simulink subsystem "nplib_sensors"  (R2024b)
settings: Solver=VariableStepAuto  StartTime=0.0  StopTime=10.0  RelTol=1e-3
undefined symbols (not defined in the file): convertTo, datetime
libraries: aerolibconvert2 x7
settings Model: Creator=CETCA  LastModifiedBy=CETCA

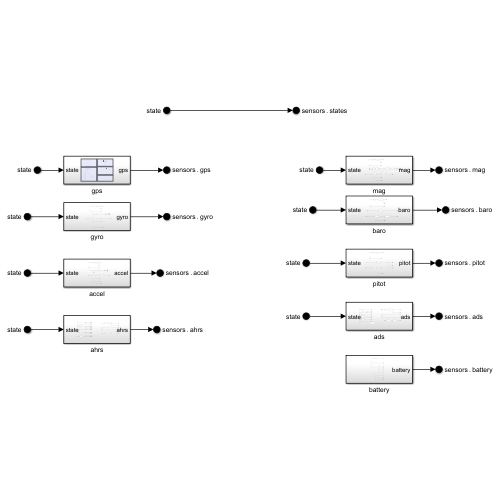
[thumbnail: Simulink's stored preview of the top-level diagram]
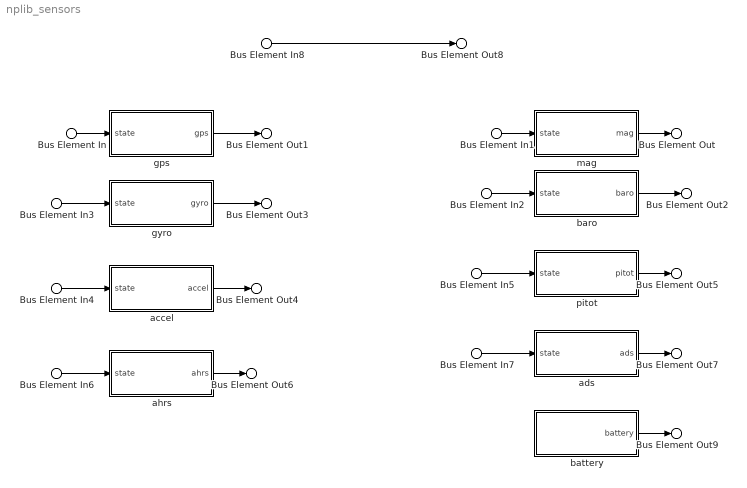
== system nplib_sensors ==
  Bus Element In{,1..8} (9 alike) : Inport  PortName=state
  accel : Subsystem
  ads : Subsystem
  ahrs : Subsystem
  baro : Subsystem
  battery : Subsystem
  gps : Subsystem
  gyro : Subsystem
  mag : Subsystem
  pitot : Subsystem
  Bus Element Out8 : Outport  PortName=sensors  Element=states
  Bus Element Out1 : Outport  PortName=sensors  Element=gps
  Bus Element Out3 : Outport  PortName=sensors  Element=gyro
  Bus Element Out : Outport  PortName=sensors  Element=mag
  Bus Element Out2 : Outport  PortName=sensors  Element=baro
  Bus Element Out5 : Outport  PortName=sensors  Element=pitot
  Bus Element Out7 : Outport  PortName=sensors  Element=ads
  Bus Element Out6 : Outport  PortName=sensors  Element=ahrs
  Bus Element Out4 : Outport  PortName=sensors  Element=accel
  Bus Element Out9 : Outport  PortName=sensors  Element=battery
  wires:
  Bus Element In7/1 -> ads/1(state)
  Bus Element In6/1 -> ahrs/1(state)
  Bus Element In8/1 -> Bus Element Out8/1
  baro/1(baro) -> Bus Element Out2/1
  Bus Element In5/1 -> pitot/1(state)
  mag/1(mag) -> Bus Element Out/1
  battery/1(battery) -> Bus Element Out9/1
  Bus Element In2/1 -> baro/1(state)
  ahrs/1(ahrs) -> Bus Element Out6/1
  Bus Element In1/1 -> mag/1(state)
  pitot/1(pitot) -> Bus Element Out5/1
  accel/1(accel) -> Bus Element Out4/1
  Bus Element In4/1 -> accel/1(state)
  gyro/1(gyro) -> Bus Element Out3/1
  Bus Element In3/1 -> gyro/1(state)
  ads/1(ads) -> Bus Element Out7/1
  Bus Element In/1 -> gps/1(state)
  gps/1(gps) -> Bus Element Out1/1

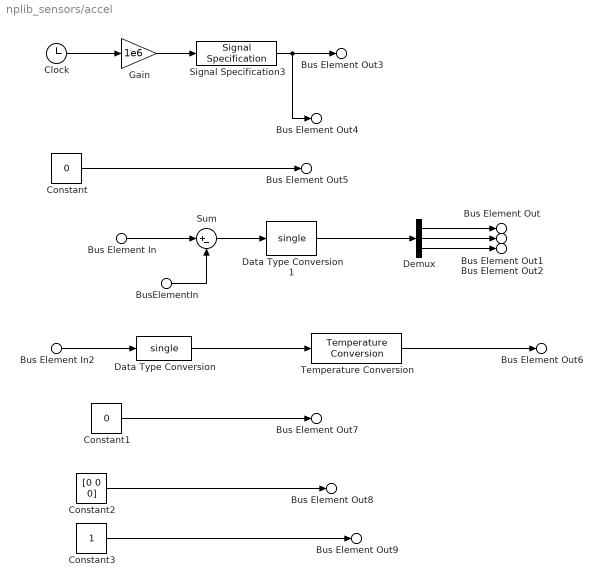
== system nplib_sensors/accel ==
  Bus Element In2 : Inport  PortName=state  Element=environ.atmosphere.temperature
  BusElementIn : Inport  PortName=state  Element=environ.gravity.gx_gy_gz
  Bus Element In : Inport  PortName=state  Element=aircraft.position.ax_ay_az
  Clock : Clock
  Constant : Constant  Value=0  OutDataTypeStr=uint32
  Constant1 : Constant  Value=0  OutDataTypeStr=uint32
  Constant2 : Constant  Value=[0 0 0]  OutDataTypeStr=uint8
  Constant3 : Constant  OutDataTypeStr=uint8
  Data Type Conversion : DataTypeConversion  OutDataTypeStr=single  SaturateOnIntegerOverflow=off  RndMeth=Floor
  Data Type Conversion1 : DataTypeConversion  OutDataTypeStr=single  SaturateOnIntegerOverflow=off  RndMeth=Floor
  Demux : Demux  Outputs=3
  Gain : Gain  Gain=1e6  OutDataTypeStr=uint64
  Signal Specification3 : SignalSpecification  Unit=µs
  Sum : Sum  Inputs=|+-
  Temperature Conversion : aerolibconvert2/Temperature Conversion  IU=K  OU=C
  Bus Element Out3 : Outport  PortName=accel  Element=timestamp
  Bus Element Out4 : Outport  PortName=accel  Element=timestamp_sample
  Bus Element Out5 : Outport  PortName=accel  Element=device_id
  Bus Element Out : Outport  PortName=accel  Element=x
  Bus Element Out1 : Outport  PortName=accel  Element=y
  Bus Element Out2 : Outport  PortName=accel  Element=z
  Bus Element Out6 : Outport  PortName=accel  Element=temperature
  Bus Element Out7 : Outport  PortName=accel  Element=error_count
  Bus Element Out8 : Outport  PortName=accel  Element=clip_counter
  Bus Element Out9 : Outport  PortName=accel  Element=samples
  wires:
  Constant3/1 -> Bus Element Out9/1
  Constant2/1 -> Bus Element Out8/1
  Demux/1 -> Bus Element Out/1
  Demux/2 -> Bus Element Out1/1
  Demux/3 -> Bus Element Out2/1
  Clock/1 -> Gain/1
  Signal Specification3/1 -> Bus Element Out4/1, Bus Element Out3/1
  Gain/1 -> Signal Specification3/1
  Constant/1 -> Bus Element Out5/1
  Constant1/1 -> Bus Element Out7/1
  Bus Element In2/1 -> Data Type Conversion/1
  Temperature Conversion/1 -> Bus Element Out6/1
  Data Type Conversion/1 -> Temperature Conversion/1
  Data Type Conversion1/1 -> Demux/1
  Bus Element In/1 -> Sum/1
  BusElementIn/1 -> Sum/2
  Sum/1 -> Data Type Conversion1/1

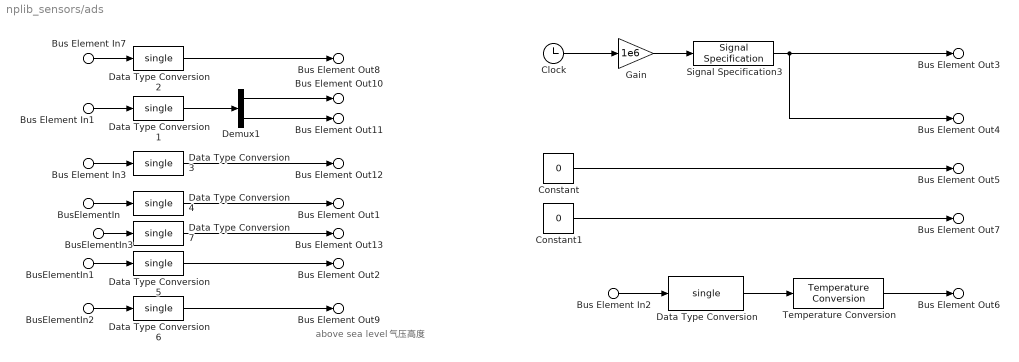
== system nplib_sensors/ads ==
  note: above sea level
      | 气压高度
  Bus Element In2 : Inport  PortName=state  Element=environ.atmosphere.temperature
  BusElementIn : Inport  PortName=state  Element=environ.atmosphere.ps
  BusElementIn1 : Inport  PortName=state  Element=environ.atmosphere.rho
  BusElementIn3 : Inport  PortName=state  Element=environ.atmosphere.pt
  Bus Element In1 : Inport  PortName=state  Element=aircraft.airdata.alpha_beta
  Bus Element In7 : Inport  PortName=state  Element=aircraft.airdata.airspeed
  Bus Element In3 : Inport  PortName=state  Element=aircraft.airdata.qbar
  BusElementIn2 : Inport  PortName=state  Element=aircraft.position.alt
  Clock : Clock
  Constant : Constant  Value=0  OutDataTypeStr=uint32
  Constant1 : Constant  Value=0  OutDataTypeStr=uint32
  Data Type Conversion{,1..7} (8 alike) : DataTypeConversion  OutDataTypeStr=single  SaturateOnIntegerOverflow=off  RndMeth=Floor
  Demux1 : Demux  Outputs=2
  Gain : Gain  Gain=1e6  OutDataTypeStr=uint64
  Signal Specification3 : SignalSpecification  Unit=µs
  Temperature Conversion : aerolibconvert2/Temperature Conversion  IU=K  OU=C
  Bus Element Out3 : Outport  PortName=ads  Element=timestamp
  Bus Element Out4 : Outport  PortName=ads  Element=timestamp_sample
  Bus Element Out5 : Outport  PortName=ads  Element=device_id
  Bus Element Out7 : Outport  PortName=ads  Element=error_count
  Bus Element Out6 : Outport  PortName=ads  Element=temperature
  Bus Element Out8 : Outport  PortName=ads  Element=va
  Bus Element Out10 : Outport  PortName=ads  Element=alpha
  Bus Element Out11 : Outport  PortName=ads  Element=beta
  Bus Element Out12 : Outport  PortName=ads  Element=qbar
  Bus Element Out13 : Outport  PortName=ads  Element=pt
  Bus Element Out1 : Outport  PortName=ads  Element=ps
  Bus Element Out2 : Outport  PortName=ads  Element=rho
  Bus Element Out9 : Outport  PortName=ads  Element=asl
  wires:
  Data Type Conversion3/1 -> Bus Element Out12/1
  Bus Element In3/1 -> Data Type Conversion3/1
  Demux1/2 -> Bus Element Out11/1
  Demux1/1 -> Bus Element Out10/1
  Bus Element In1/1 -> Data Type Conversion1/1
  Clock/1 -> Gain/1
  Signal Specification3/1 -> Bus Element Out4/1, Bus Element Out3/1
  Gain/1 -> Signal Specification3/1
  Constant/1 -> Bus Element Out5/1
  Constant1/1 -> Bus Element Out7/1
  Bus Element In2/1 -> Data Type Conversion/1
  Temperature Conversion/1 -> Bus Element Out6/1
  Data Type Conversion/1 -> Temperature Conversion/1
  Bus Element In7/1 -> Data Type Conversion2/1
  Data Type Conversion1/1 -> Demux1/1
  Data Type Conversion2/1 -> Bus Element Out8/1
  BusElementIn/1 -> Data Type Conversion4/1
  Data Type Conversion4/1 -> Bus Element Out1/1
  BusElementIn1/1 -> Data Type Conversion5/1
  Data Type Conversion5/1 -> Bus Element Out2/1
  BusElementIn2/1 -> Data Type Conversion6/1
  Data Type Conversion6/1 -> Bus Element Out9/1
  Data Type Conversion7/1 -> Bus Element Out13/1
  BusElementIn3/1 -> Data Type Conversion7/1

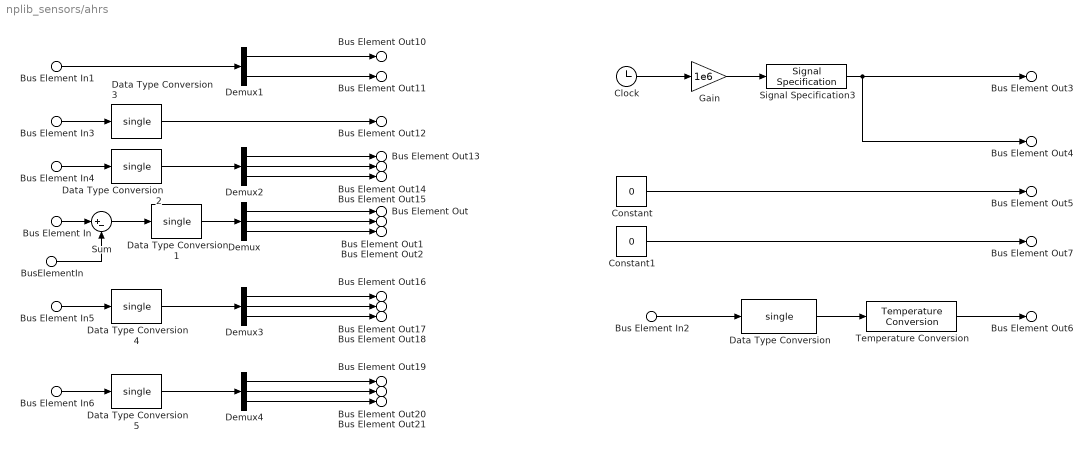
== system nplib_sensors/ahrs ==
  Bus Element In2 : Inport  PortName=state  Element=environ.atmosphere.temperature
  BusElementIn : Inport  PortName=state  Element=environ.gravity.gx_gy_gz
  Bus Element In : Inport  PortName=state  Element=aircraft.position.ax_ay_az
  Bus Element In1 : Inport  PortName=state  Element=aircraft.position.lat_lon
  Bus Element In3 : Inport  PortName=state  Element=aircraft.position.alt
  Bus Element In4 : Inport  PortName=state  Element=aircraft.position.vn_ve_vd
  Bus Element In5 : Inport  PortName=state  Element=aircraft.attitude.phi_theta_psi
  Bus Element In6 : Inport  PortName=state  Element=aircraft.attitude.p_q_r
  Clock : Clock
  Constant : Constant  Value=0  OutDataTypeStr=uint32
  Constant1 : Constant  Value=0  OutDataTypeStr=uint32
  Data Type Conversion{,1..5} (6 alike) : DataTypeConversion  OutDataTypeStr=single  SaturateOnIntegerOverflow=off  RndMeth=Floor
  Demux{,2..4} (4 alike) : Demux  Outputs=3
  Demux1 : Demux  Outputs=2
  Gain : Gain  Gain=1e6  OutDataTypeStr=uint64
  Signal Specification3 : SignalSpecification  Unit=µs
  Sum : Sum  Inputs=|+-
  Temperature Conversion : aerolibconvert2/Temperature Conversion  IU=K  OU=C
  Bus Element Out3 : Outport  PortName=ahrs  Element=timestamp
  Bus Element Out4 : Outport  PortName=ahrs  Element=timestamp_sample
  Bus Element Out5 : Outport  PortName=ahrs  Element=device_id
  Bus Element Out7 : Outport  PortName=ahrs  Element=error_count
  Bus Element Out6 : Outport  PortName=ahrs  Element=temperature
  Bus Element Out10 : Outport  PortName=ahrs  Element=lat
  Bus Element Out11 : Outport  PortName=ahrs  Element=lon
  Bus Element Out12 : Outport  PortName=ahrs  Element=alt
  Bus Element Out13 : Outport  PortName=ahrs  Element=vn
  Bus Element Out14 : Outport  PortName=ahrs  Element=ve
  Bus Element Out15 : Outport  PortName=ahrs  Element=vd
  Bus Element Out : Outport  PortName=ahrs  Element=ax
  Bus Element Out1 : Outport  PortName=ahrs  Element=ay
  Bus Element Out2 : Outport  PortName=ahrs  Element=az
  Bus Element Out16 : Outport  PortName=ahrs  Element=phi
  Bus Element Out17 : Outport  PortName=ahrs  Element=theta
  Bus Element Out18 : Outport  PortName=ahrs  Element=psi
  Bus Element Out19 : Outport  PortName=ahrs  Element=p
  Bus Element Out20 : Outport  PortName=ahrs  Element=q
  Bus Element Out21 : Outport  PortName=ahrs  Element=r
  wires:
  Data Type Conversion1/1 -> Demux/1
  Data Type Conversion/1 -> Temperature Conversion/1
  Temperature Conversion/1 -> Bus Element Out6/1
  Bus Element In2/1 -> Data Type Conversion/1
  Constant1/1 -> Bus Element Out7/1
  Constant/1 -> Bus Element Out5/1
  Gain/1 -> Signal Specification3/1
  Signal Specification3/1 -> Bus Element Out3/1, Bus Element Out4/1
  Clock/1 -> Gain/1
  Demux/3 -> Bus Element Out2/1
  Demux/2 -> Bus Element Out1/1
  Demux/1 -> Bus Element Out/1
  Bus Element In1/1 -> Demux1/1
  Demux1/1 -> Bus Element Out10/1
  Demux1/2 -> Bus Element Out11/1
  Bus Element In3/1 -> Data Type Conversion3/1
  Bus Element In4/1 -> Data Type Conversion2/1
  Demux2/1 -> Bus Element Out13/1
  Demux2/2 -> Bus Element Out14/1
  Demux2/3 -> Bus Element Out15/1
  Bus Element In5/1 -> Data Type Conversion4/1
  Demux3/1 -> Bus Element Out16/1
  Demux3/2 -> Bus Element Out17/1
  Demux3/3 -> Bus Element Out18/1
  Bus Element In6/1 -> Data Type Conversion5/1
  Demux4/1 -> Bus Element Out19/1
  Demux4/2 -> Bus Element Out20/1
  Demux4/3 -> Bus Element Out21/1
  Data Type Conversion2/1 -> Demux2/1
  Data Type Conversion3/1 -> Bus Element Out12/1
  Data Type Conversion4/1 -> Demux3/1
  Data Type Conversion5/1 -> Demux4/1
  Bus Element In/1 -> Sum/1
  Sum/1 -> Data Type Conversion1/1
  BusElementIn/1 -> Sum/2

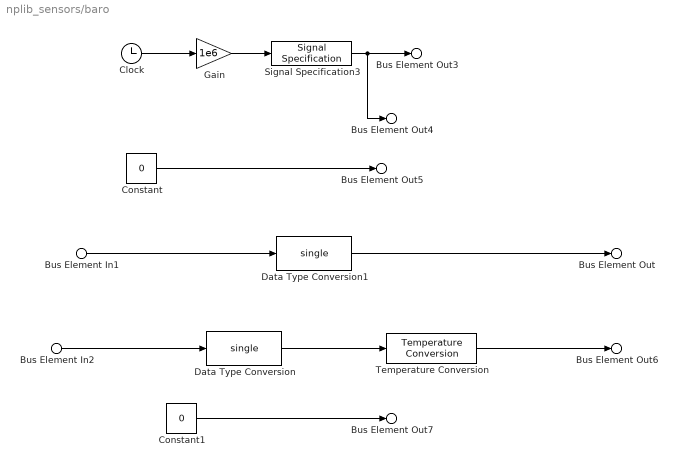
== system nplib_sensors/baro ==
  Bus Element In2 : Inport  PortName=state  Element=environ.atmosphere.temperature
  Bus Element In1 : Inport  PortName=state  Element=environ.atmosphere.ps
  Clock : Clock
  Constant : Constant  Value=0  OutDataTypeStr=uint32
  Constant1 : Constant  Value=0  OutDataTypeStr=uint32
  Data Type Conversion : DataTypeConversion  OutDataTypeStr=single  SaturateOnIntegerOverflow=off  RndMeth=Floor
  Data Type Conversion1 : DataTypeConversion  OutDataTypeStr=single  SaturateOnIntegerOverflow=off  RndMeth=Floor
  Gain : Gain  Gain=1e6  OutDataTypeStr=uint64
  Signal Specification3 : SignalSpecification  Unit=µs
  Temperature Conversion : aerolibconvert2/Temperature Conversion  IU=K  OU=C
  Bus Element Out3 : Outport  PortName=baro  Element=timestamp
  Bus Element Out4 : Outport  PortName=baro  Element=timestamp_sample
  Bus Element Out5 : Outport  PortName=baro  Element=device_id
  Bus Element Out7 : Outport  PortName=baro  Element=error_count
  Bus Element Out : Outport  PortName=baro  Element=pressure
  Bus Element Out6 : Outport  PortName=baro  Element=temperature
  wires:
  Clock/1 -> Gain/1
  Signal Specification3/1 -> Bus Element Out4/1, Bus Element Out3/1
  Gain/1 -> Signal Specification3/1
  Constant/1 -> Bus Element Out5/1
  Constant1/1 -> Bus Element Out7/1
  Bus Element In2/1 -> Data Type Conversion/1
  Temperature Conversion/1 -> Bus Element Out6/1
  Data Type Conversion/1 -> Temperature Conversion/1
  Bus Element In1/1 -> Data Type Conversion1/1
  Data Type Conversion1/1 -> Bus Element Out/1

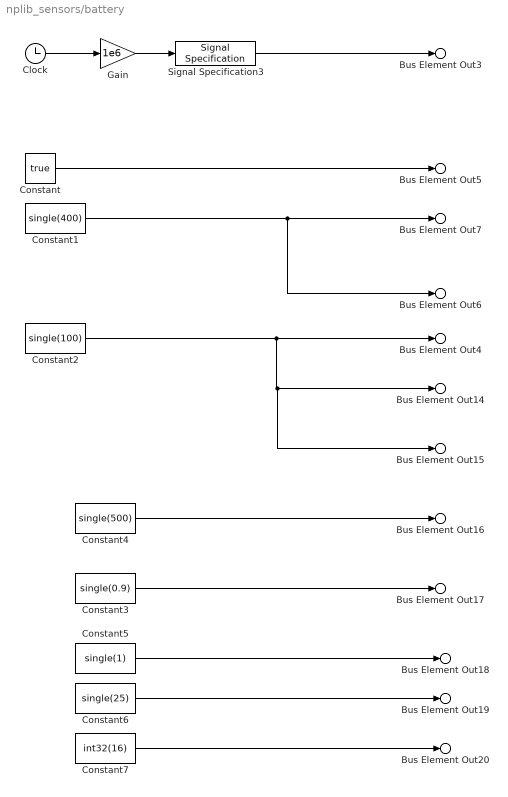
== system nplib_sensors/battery ==
  Clock : Clock
  Constant : Constant  Value=true
  Constant1 : Constant  Value=single(400)
  Constant2 : Constant  Value=single(100)
  Constant3 : Constant  Value=single(0.9)
  Constant4 : Constant  Value=single(500)
  Constant5 : Constant  Value=single(1)
  Constant6 : Constant  Value=single(25)
  Constant7 : Constant  Value=int32(16)
  Gain : Gain  Gain=1e6  OutDataTypeStr=uint64
  Signal Specification3 : SignalSpecification  Unit=µs
  Bus Element Out3 : Outport  PortName=battery  Element=timestamp
  Bus Element Out5 : Outport  PortName=battery  Element=connected
  Bus Element Out7 : Outport  PortName=battery  Element=voltage_v
  Bus Element Out6 : Outport  PortName=battery  Element=voltage_filtered_v
  Bus Element Out4 : Outport  PortName=battery  Element=current_a
  Bus Element Out14 : Outport  PortName=battery  Element=current_filtered_a
  Bus Element Out15 : Outport  PortName=battery  Element=current_average_a
  Bus Element Out16 : Outport  PortName=battery  Element=discharged_mah
  Bus Element Out17 : Outport  PortName=battery  Element=remaining
  Bus Element Out18 : Outport  PortName=battery  Element=scale
  Bus Element Out19 : Outport  PortName=battery  Element=temperature
  Bus Element Out20 : Outport  PortName=battery  Element=cell_count
  wires:
  Constant1/1 -> Bus Element Out6/1, Bus Element Out7/1
  Constant/1 -> Bus Element Out5/1
  Gain/1 -> Signal Specification3/1
  Signal Specification3/1 -> Bus Element Out3/1
  Clock/1 -> Gain/1
  Constant2/1 -> Bus Element Out15/1, Bus Element Out14/1, Bus Element Out4/1
  Constant3/1 -> Bus Element Out17/1
  Constant4/1 -> Bus Element Out16/1
  Constant5/1 -> Bus Element Out18/1
  Constant6/1 -> Bus Element Out19/1
  Constant7/1 -> Bus Element Out20/1

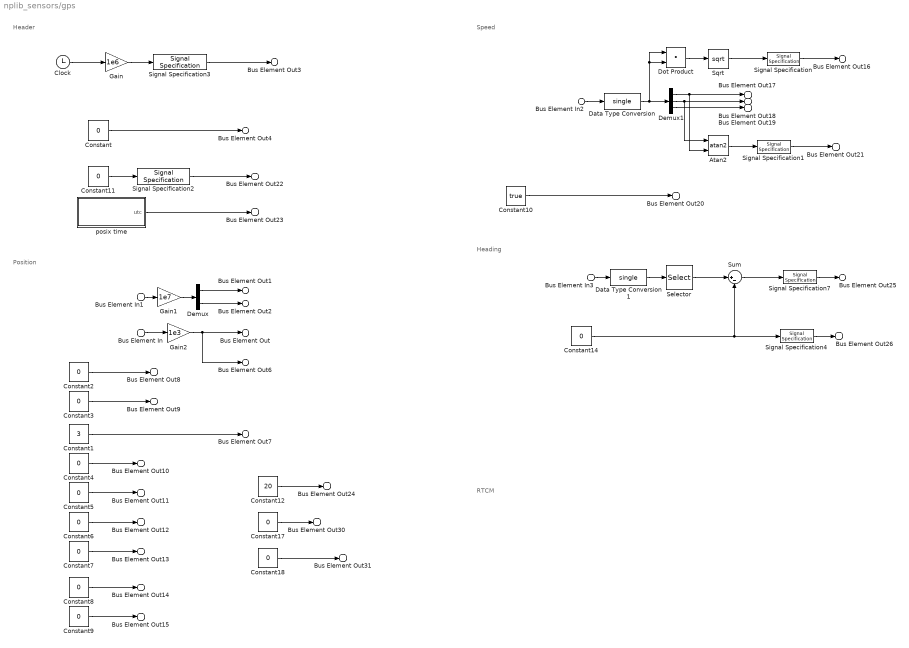
== system nplib_sensors/gps ==
  note: RTCM
  note: Heading
  note: Speed
  note: Header
  note: Position
  Bus Element In : Inport  PortName=state  Element=aircraft.position.alt
  Bus Element In1 : Inport  PortName=state  Element=aircraft.position.lat_lon
  Bus Element In2 : Inport  PortName=state  Element=aircraft.position.vn_ve_vd
  Bus Element In3 : Inport  PortName=state  Element=aircraft.attitude.phi_theta_psi
  Atan2 : Trigonometry  Operator=atan2
  Clock : Clock
  Constant : Constant  Value=0  OutDataTypeStr=uint32
  Constant1 : Constant  Value=3  OutDataTypeStr=uint8
  Constant10 : Constant  Value=true  OutDataTypeStr=boolean
  Constant11 : Constant  Value=0  OutDataTypeStr=int32
  Constant12 : Constant  Value=20  OutDataTypeStr=uint8
  Constant{2..7,14} (7 alike) : Constant  Value=0  OutDataTypeStr=single
  Constant17 : Constant  Value=0  OutDataTypeStr=uint8
  Constant18 : Constant  Value=0  OutDataTypeStr=int32
  Constant8 : Constant  Value=0  OutDataTypeStr=int32
  Constant9 : Constant  Value=0  OutDataTypeStr=uint16
  Data Type Conversion : DataTypeConversion  OutDataTypeStr=single  SaturateOnIntegerOverflow=off  RndMeth=Floor
  Data Type Conversion1 : DataTypeConversion  OutDataTypeStr=single  SaturateOnIntegerOverflow=off  RndMeth=Floor
  Demux : Demux  Outputs=2
  Demux1 : Demux  Outputs=3
  Dot Product : DotProduct  OutDataTypeStr=Inherit: Inherit via internal rule
  Gain : Gain  Gain=1e6  OutDataTypeStr=uint64
  Gain1 : Gain  Gain=1e7  OutDataTypeStr=int32
  Gain2 : Gain  Gain=1e3  OutDataTypeStr=int32
  Selector : Selector  InputPortWidth=3  IndexOptions=Index vector (dialog)  Indices=3  OutputSizes=1
  Signal Specification : SignalSpecification  Unit=m/s
  Signal Specification1 : SignalSpecification  Unit=rad
  Signal Specification2 : SignalSpecification  Unit=ms
  Signal Specification3 : SignalSpecification  Unit=µs
  Signal Specification4 : SignalSpecification  Unit=rad
  Signal Specification7 : SignalSpecification  Unit=rad
  Sqrt : Sqrt
  Sum : Sum  Inputs=|+-
  posix time : Subsystem
  Bus Element Out3 : Outport  PortName=gps  Element=timestamp
  Bus Element Out4 : Outport  PortName=gps  Element=device_id
  Bus Element Out1 : Outport  PortName=gps  Element=lat
  Bus Element Out2 : Outport  PortName=gps  Element=lon
  Bus Element Out : Outport  PortName=gps  Element=alt
  Bus Element Out6 : Outport  PortName=gps  Element=alt_ellipsoid
  Bus Element Out8 : Outport  PortName=gps  Element=s_variance_m_s
  Bus Element Out9 : Outport  PortName=gps  Element=c_variance_rad
  Bus Element Out7 : Outport  PortName=gps  Element=fix_type
  Bus Element Out10 : Outport  PortName=gps  Element=eph
  Bus Element Out11 : Outport  PortName=gps  Element=epv
  Bus Element Out12 : Outport  PortName=gps  Element=hdop
  Bus Element Out13 : Outport  PortName=gps  Element=vdop
  Bus Element Out14 : Outport  PortName=gps  Element=noise_per_ms
  Bus Element Out15 : Outport  PortName=gps  Element=automatic_gain_control
  Bus Element Out31 : Outport  PortName=gps  Element=jamming_indicator
  Bus Element Out30 : Outport  PortName=gps  Element=jamming_state
  Bus Element Out16 : Outport  PortName=gps  Element=vel_m_s
  Bus Element Out17 : Outport  PortName=gps  Element=vel_n_m_s
  Bus Element Out18 : Outport  PortName=gps  Element=vel_e_m_s
  Bus Element Out19 : Outport  PortName=gps  Element=vel_d_m_s
  Bus Element Out21 : Outport  PortName=gps  Element=cog_rad
  Bus Element Out20 : Outport  PortName=gps  Element=vel_ned_valid
  Bus Element Out22 : Outport  PortName=gps  Element=timestamp_time_relative
  Bus Element Out23 : Outport  PortName=gps  Element=time_utc_usec
  Bus Element Out24 : Outport  PortName=gps  Element=satellites_used
  Bus Element Out25 : Outport  PortName=gps  Element=heading
  Bus Element Out26 : Outport  PortName=gps  Element=heading_offset
  wires:
  Bus Element In/1 -> Gain2/1
  Bus Element In1/1 -> Gain1/1
  Demux/1 -> Bus Element Out1/1
  Demux/2 -> Bus Element Out2/1
  Clock/1 -> Gain/1
  Gain/1 -> Signal Specification3/1
  Constant/1 -> Bus Element Out4/1
  Gain1/1 -> Demux/1
  Gain2/1 -> Bus Element Out6/1, Bus Element Out/1
  Constant1/1 -> Bus Element Out7/1
  Constant2/1 -> Bus Element Out8/1
  Constant3/1 -> Bus Element Out9/1
  Constant4/1 -> Bus Element Out10/1
  Constant5/1 -> Bus Element Out11/1
  Constant7/1 -> Bus Element Out13/1
  Constant6/1 -> Bus Element Out12/1
  Constant9/1 -> Bus Element Out15/1
  Constant8/1 -> Bus Element Out14/1
  Bus Element In2/1 -> Data Type Conversion/1
  Demux1/1 -> Atan2/2, Bus Element Out17/1
  Demux1/2 -> Atan2/1, Bus Element Out18/1
  Demux1/3 -> Bus Element Out19/1
  Constant10/1 -> Bus Element Out20/1
  Atan2/1 -> Signal Specification1/1
  Sqrt/1 -> Signal Specification/1
  Dot Product/1 -> Sqrt/1
  Data Type Conversion/1 -> Demux1/1, Dot Product/1, Dot Product/2
  Signal Specification/1 -> Bus Element Out16/1
  Signal Specification1/1 -> Bus Element Out21/1
  Constant12/1 -> Bus Element Out24/1
  Bus Element In3/1 -> Data Type Conversion1/1
  Constant14/1 -> Sum/2, Signal Specification4/1
  Selector/1 -> Sum/1
  Sum/1 -> Signal Specification7/1
  Constant11/1 -> Signal Specification2/1
  posix time/1(utc) -> Bus Element Out23/1
  Signal Specification2/1 -> Bus Element Out22/1
  Signal Specification3/1 -> Bus Element Out3/1
  Signal Specification4/1 -> Bus Element Out26/1
  Constant17/1 -> Bus Element Out30/1
  Constant18/1 -> Bus Element Out31/1
  Signal Specification7/1 -> Bus Element Out25/1
  Data Type Conversion1/1 -> Selector/1

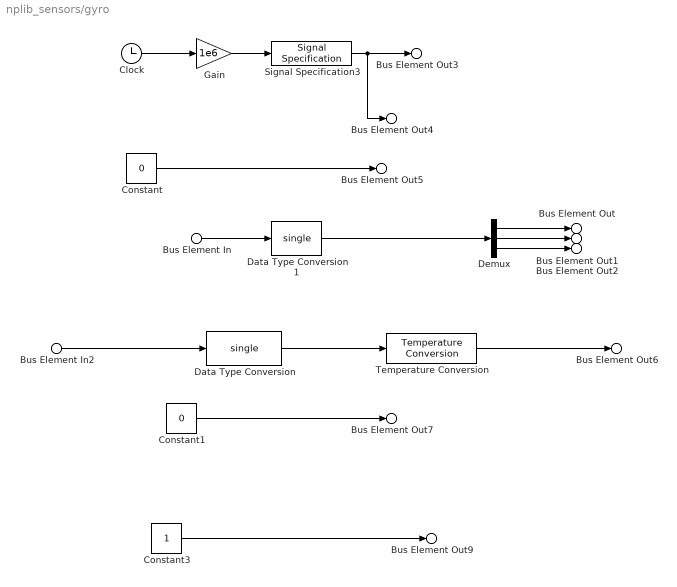
== system nplib_sensors/gyro ==
  Bus Element In2 : Inport  PortName=state  Element=environ.atmosphere.temperature
  Bus Element In : Inport  PortName=state  Element=aircraft.attitude.p_q_r
  Clock : Clock
  Constant : Constant  Value=0  OutDataTypeStr=uint32
  Constant1 : Constant  Value=0  OutDataTypeStr=uint32
  Constant3 : Constant  OutDataTypeStr=uint8
  Data Type Conversion : DataTypeConversion  OutDataTypeStr=single  SaturateOnIntegerOverflow=off  RndMeth=Floor
  Data Type Conversion1 : DataTypeConversion  OutDataTypeStr=single  SaturateOnIntegerOverflow=off  RndMeth=Floor
  Demux : Demux  Outputs=3
  Gain : Gain  Gain=1e6  OutDataTypeStr=uint64
  Signal Specification3 : SignalSpecification  Unit=µs
  Temperature Conversion : aerolibconvert2/Temperature Conversion  IU=K  OU=C
  Bus Element Out3 : Outport  PortName=gyro  Element=timestamp
  Bus Element Out4 : Outport  PortName=gyro  Element=timestamp_sample
  Bus Element Out5 : Outport  PortName=gyro  Element=device_id
  Bus Element Out : Outport  PortName=gyro  Element=x
  Bus Element Out1 : Outport  PortName=gyro  Element=y
  Bus Element Out2 : Outport  PortName=gyro  Element=z
  Bus Element Out6 : Outport  PortName=gyro  Element=temperature
  Bus Element Out7 : Outport  PortName=gyro  Element=error_count
  Bus Element Out9 : Outport  PortName=gyro  Element=samples
  wires:
  Data Type Conversion1/1 -> Demux/1
  Data Type Conversion/1 -> Temperature Conversion/1
  Temperature Conversion/1 -> Bus Element Out6/1
  Bus Element In2/1 -> Data Type Conversion/1
  Constant1/1 -> Bus Element Out7/1
  Constant/1 -> Bus Element Out5/1
  Gain/1 -> Signal Specification3/1
  Signal Specification3/1 -> Bus Element Out3/1, Bus Element Out4/1
  Clock/1 -> Gain/1
  Demux/3 -> Bus Element Out2/1
  Demux/2 -> Bus Element Out1/1
  Demux/1 -> Bus Element Out/1
  Bus Element In/1 -> Data Type Conversion1/1
  Constant3/1 -> Bus Element Out9/1

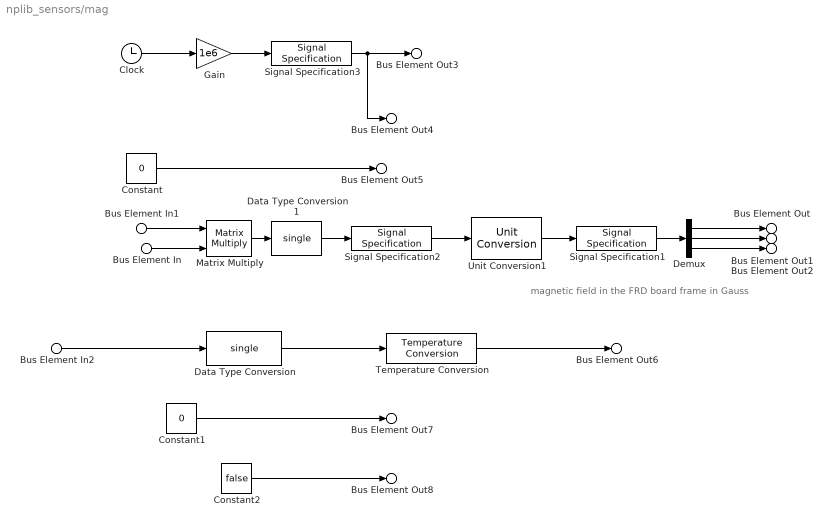
== system nplib_sensors/mag ==
  note: magnetic field in the FRD board frame in Gauss
  Bus Element In : Inport  PortName=state  Element=environ.magnetic.xyz
  Bus Element In2 : Inport  PortName=state  Element=environ.atmosphere.temperature
  Bus Element In1 : Inport  PortName=state  Element=aircraft.attitude.Rbe
  Clock : Clock
  Constant : Constant  Value=0  OutDataTypeStr=uint32
  Constant1 : Constant  Value=0  OutDataTypeStr=uint32
  Constant2 : Constant  Value=false
  Data Type Conversion : DataTypeConversion  OutDataTypeStr=single  SaturateOnIntegerOverflow=off  RndMeth=Floor
  Data Type Conversion1 : DataTypeConversion  OutDataTypeStr=single  SaturateOnIntegerOverflow=off  RndMeth=Floor
  Demux : Demux  Outputs=3
  Gain : Gain  Gain=1e6  OutDataTypeStr=uint64
  Matrix Multiply : Product  Multiplication=Matrix(*)
  Signal Specification1 : SignalSpecification  Unit=G
  Signal Specification2 : SignalSpecification  Unit=nT
  Signal Specification3 : SignalSpecification  Unit=µs
  Temperature Conversion : aerolibconvert2/Temperature Conversion  IU=K  OU=C
  Unit Conversion1 : UnitConversion
  Bus Element Out3 : Outport  PortName=mag  Element=timestamp
  Bus Element Out4 : Outport  PortName=mag  Element=timestamp_sample
  Bus Element Out5 : Outport  PortName=mag  Element=device_id
  Bus Element Out : Outport  PortName=mag  Element=x
  Bus Element Out1 : Outport  PortName=mag  Element=y
  Bus Element Out2 : Outport  PortName=mag  Element=z
  Bus Element Out6 : Outport  PortName=mag  Element=temperature
  Bus Element Out7 : Outport  PortName=mag  Element=error_count
  Bus Element Out8 : Outport  PortName=mag  Element=is_external
  wires:
  Bus Element In/1 -> Matrix Multiply/2
  Bus Element In1/1 -> Matrix Multiply/1
  Matrix Multiply/1 -> Data Type Conversion1/1
  Demux/1 -> Bus Element Out/1
  Demux/2 -> Bus Element Out1/1
  Demux/3 -> Bus Element Out2/1
  Clock/1 -> Gain/1
  Signal Specification3/1 -> Bus Element Out4/1, Bus Element Out3/1
  Gain/1 -> Signal Specification3/1
  Constant/1 -> Bus Element Out5/1
  Constant1/1 -> Bus Element Out7/1
  Bus Element In2/1 -> Data Type Conversion/1
  Temperature Conversion/1 -> Bus Element Out6/1
  Data Type Conversion/1 -> Temperature Conversion/1
  Data Type Conversion1/1 -> Signal Specification2/1
  Signal Specification1/1 -> Demux/1
  Unit Conversion1/1 -> Signal Specification1/1
  Signal Specification2/1 -> Unit Conversion1/1
  Constant2/1 -> Bus Element Out8/1

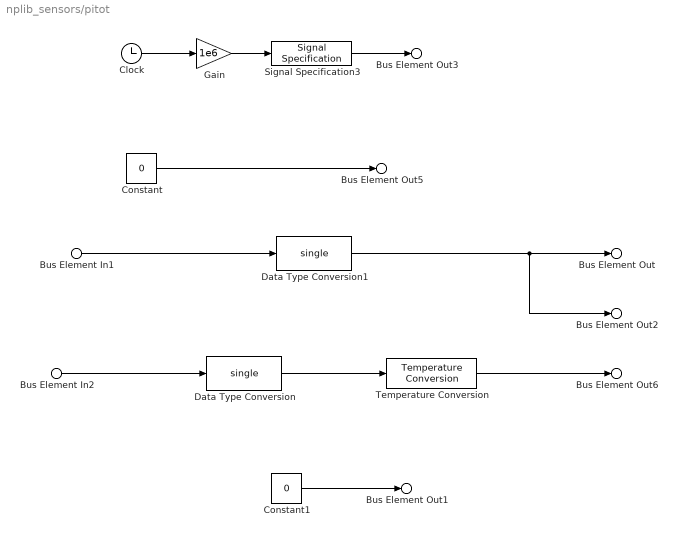
== system nplib_sensors/pitot ==
  Bus Element In2 : Inport  PortName=state  Element=environ.atmosphere.temperature
  Bus Element In1 : Inport  PortName=state  Element=aircraft.airdata.qbar
  Clock : Clock
  Constant : Constant  Value=0  OutDataTypeStr=uint32
  Constant1 : Constant  Value=0  OutDataTypeStr=uint64
  Data Type Conversion : DataTypeConversion  OutDataTypeStr=single  SaturateOnIntegerOverflow=off  RndMeth=Floor
  Data Type Conversion1 : DataTypeConversion  OutDataTypeStr=single  SaturateOnIntegerOverflow=off  RndMeth=Floor
  Gain : Gain  Gain=1e6  OutDataTypeStr=uint64
  Signal Specification3 : SignalSpecification  Unit=µs
  Temperature Conversion : aerolibconvert2/Temperature Conversion  IU=K  OU=C
  Bus Element Out3 : Outport  PortName=pitot  Element=timestamp
  Bus Element Out1 : Outport  PortName=pitot  Element=error_count
  Bus Element Out : Outport  PortName=pitot  Element=differential_pressure_raw_pa
  Bus Element Out2 : Outport  PortName=pitot  Element=differential_pressure_filtered_pa
  Bus Element Out6 : Outport  PortName=pitot  Element=temperature
  Bus Element Out5 : Outport  PortName=pitot  Element=device_id
  wires:
  Data Type Conversion1/1 -> Bus Element Out2/1, Bus Element Out/1
  Bus Element In1/1 -> Data Type Conversion1/1
  Data Type Conversion/1 -> Temperature Conversion/1
  Temperature Conversion/1 -> Bus Element Out6/1
  Bus Element In2/1 -> Data Type Conversion/1
  Constant/1 -> Bus Element Out5/1
  Gain/1 -> Signal Specification3/1
  Signal Specification3/1 -> Bus Element Out3/1
  Clock/1 -> Gain/1
  Constant1/1 -> Bus Element Out1/1

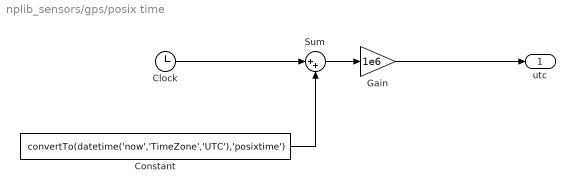
== system nplib_sensors/gps/posix time ==
  Clock : Clock
  Constant : Constant  Value=convertTo(datetime('now','TimeZone','UTC'),'posixtime')
  Gain : Gain  Gain=1e6  OutDataTypeStr=uint64
  Sum : Sum  Inputs=|++
  utc : Outport  Unit=µs
  wires:
  Clock/1 -> Sum/1
  Sum/1 -> Gain/1
  Constant/1 -> Sum/2
  Gain/1 -> utc/1
